simulink model "Delta_Model_Separate"  (R2023a)
settings: Solver=VariableStepAuto  StartTime=0.0  StopTime=10.0  RelTol=1e-3
values from neighbouring files (symbols this model uses):
  coord = [start_coord carry_coord end_coord]    [calculations.m]
  dl = 0.04    [calculations.m]
  l1 = 1    [calculations.m]
  l2 = 3    [calculations.m]
  phi0 = acos((l1+r0-re)/l2)    [calculations.m]
  r0 = 1    [calculations.m]
  re = 0.2    [calculations.m]
  result_t = [start_t carry_t end_t]    [calculations.m]
undefined symbols (not defined in the file or in its folder): B, m1_1, Spline, X, Y, Z
libraries: sm_lib x109, nesl_utility x10, robotcorelib x1
(part 4 of 4)

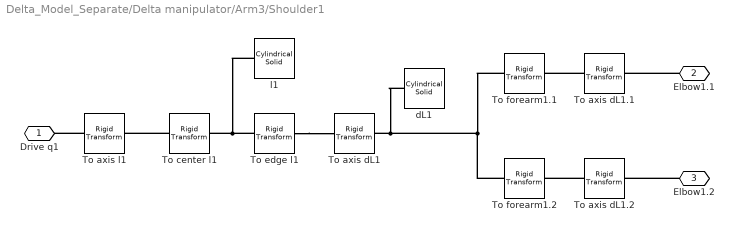
== system Delta_Model_Separate/Delta manipulator/Arm3/Shoulder1 ==
  To axis dL1 : sm_lib/Frames and Transforms/Rigid Transform  TranslationMethod=None  TranslationStandardOffset=0  TranslationStandardOffsetUnits=m  TranslationStandardAxis=+Z  TranslationCartesianOffset=[r0 0 0]  TranslationCartesianOffsetUnits=m  TranslationROffset=0  TranslationROffsetUnits=m  TranslationZOffset=0  TranslationZOffsetUnits=m  TranslationThetaOffset=0  TranslationThetaOffsetUnits=deg  RotationMethod=StandardAxis  RotationAngleUnits=rad  RotationStandardAxis=+Y  RotationAngle=pi/2  RotationArbitraryAxis=[0 0 1]  FollAlignAxisA=+X  BaseAlignAxisA=+Y  FollAlignAxisB=+Y  BaseAlignAxisB=+Z  RotationSequenceAxes=FollowerAxes  RotationSequence=XYX  RotationSequenceAngles=[0 0 0]  RotationSequenceAnglesUnits=deg  RotationMatrix=[1 0 0; 0 1 0; 0 0 1]  Quaternion=[1 0 0 0]
  To axis dL1.1 : sm_lib/Frames and Transforms/Rigid Transform  TranslationMethod=None  TranslationStandardOffset=0  TranslationStandardOffsetUnits=m  TranslationStandardAxis=+Z  TranslationCartesianOffset=[r0 0 0]  TranslationCartesianOffsetUnits=m  TranslationROffset=0  TranslationROffsetUnits=m  TranslationZOffset=0  TranslationZOffsetUnits=m  TranslationThetaOffset=0  TranslationThetaOffsetUnits=deg  RotationMethod=StandardAxis  RotationAngleUnits=rad  RotationStandardAxis=-Y  RotationAngle=pi/2  RotationArbitraryAxis=[0 0 1]  FollAlignAxisA=+X  BaseAlignAxisA=+Y  FollAlignAxisB=+Y  BaseAlignAxisB=+Z  RotationSequenceAxes=FollowerAxes  RotationSequence=XYX  RotationSequenceAngles=[0 0 0]  RotationSequenceAnglesUnits=deg  RotationMatrix=[1 0 0; 0 1 0; 0 0 1]  Quaternion=[1 0 0 0]
  To axis dL1.2 : sm_lib/Frames and Transforms/Rigid Transform  TranslationMethod=None  TranslationStandardOffset=0  TranslationStandardOffsetUnits=m  TranslationStandardAxis=+Z  TranslationCartesianOffset=[r0 0 0]  TranslationCartesianOffsetUnits=m  TranslationROffset=0  TranslationROffsetUnits=m  TranslationZOffset=0  TranslationZOffsetUnits=m  TranslationThetaOffset=0  TranslationThetaOffsetUnits=deg  RotationMethod=StandardAxis  RotationAngleUnits=rad  RotationStandardAxis=-Y  RotationAngle=pi/2  RotationArbitraryAxis=[0 0 1]  FollAlignAxisA=+X  BaseAlignAxisA=+Y  FollAlignAxisB=+Y  BaseAlignAxisB=+Z  RotationSequenceAxes=FollowerAxes  RotationSequence=XYX  RotationSequenceAngles=[0 0 0]  RotationSequenceAnglesUnits=deg  RotationMatrix=[1 0 0; 0 1 0; 0 0 1]  Quaternion=[1 0 0 0]
  To axis l1 : sm_lib/Frames and Transforms/Rigid Transform  TranslationMethod=None  TranslationStandardOffset=0  TranslationStandardOffsetUnits=m  TranslationStandardAxis=+Z  TranslationCartesianOffset=[r0 0 0]  TranslationCartesianOffsetUnits=m  TranslationROffset=0  TranslationROffsetUnits=m  TranslationZOffset=0  TranslationZOffsetUnits=m  TranslationThetaOffset=0  TranslationThetaOffsetUnits=deg  RotationMethod=StandardAxis  RotationAngleUnits=deg  RotationStandardAxis=+Y  RotationAngle=90  RotationArbitraryAxis=[0 0 1]  FollAlignAxisA=+X  BaseAlignAxisA=+Y  FollAlignAxisB=+Y  BaseAlignAxisB=+Z  RotationSequenceAxes=FollowerAxes  RotationSequence=XYX  RotationSequenceAngles=[0 0 0]  RotationSequenceAnglesUnits=deg  RotationMatrix=[1 0 0; 0 1 0; 0 0 1]  Quaternion=[1 0 0 0]
  To center l1 : sm_lib/Frames and Transforms/Rigid Transform  TranslationMethod=Cartesian  TranslationStandardOffset=0  TranslationStandardOffsetUnits=m  TranslationStandardAxis=+Z  TranslationCartesianOffset=[0 0 l1/2]  TranslationCartesianOffsetUnits=m  TranslationROffset=0  TranslationROffsetUnits=m  TranslationZOffset=0  TranslationZOffsetUnits=m  TranslationThetaOffset=0  TranslationThetaOffsetUnits=deg  RotationMethod=None  RotationAngleUnits=deg  RotationStandardAxis=+Y  RotationAngle=90  RotationArbitraryAxis=[0 0 1]  FollAlignAxisA=+X  BaseAlignAxisA=+Y  FollAlignAxisB=+Y  BaseAlignAxisB=+Z  RotationSequenceAxes=FollowerAxes  RotationSequence=XYX  RotationSequenceAngles=[0 0 0]  RotationSequenceAnglesUnits=deg  RotationMatrix=[1 0 0; 0 1 0; 0 0 1]  Quaternion=[1 0 0 0]
  To edge l1 : sm_lib/Frames and Transforms/Rigid Transform  TranslationMethod=Cartesian  TranslationStandardOffset=0  TranslationStandardOffsetUnits=m  TranslationStandardAxis=+Z  TranslationCartesianOffset=[0 0 l1/2]  TranslationCartesianOffsetUnits=m  TranslationROffset=0  TranslationROffsetUnits=m  TranslationZOffset=0  TranslationZOffsetUnits=m  TranslationThetaOffset=0  TranslationThetaOffsetUnits=deg  RotationMethod=None  RotationAngleUnits=deg  RotationStandardAxis=+Y  RotationAngle=90  RotationArbitraryAxis=[0 0 1]  FollAlignAxisA=+X  BaseAlignAxisA=+Y  FollAlignAxisB=+Y  BaseAlignAxisB=+Z  RotationSequenceAxes=FollowerAxes  RotationSequence=XYX  RotationSequenceAngles=[0 0 0]  RotationSequenceAnglesUnits=deg  RotationMatrix=[1 0 0; 0 1 0; 0 0 1]  Quaternion=[1 0 0 0]
  "To forearm1.1 " : sm_lib/Frames and Transforms/Rigid Transform  TranslationMethod=Cartesian  TranslationStandardOffset=0  TranslationStandardOffsetUnits=m  TranslationStandardAxis=+Z  TranslationCartesianOffset=[0 0 dl/2]  TranslationCartesianOffsetUnits=m  TranslationROffset=0  TranslationROffsetUnits=m  TranslationZOffset=0  TranslationZOffsetUnits=m  TranslationThetaOffset=0  TranslationThetaOffsetUnits=deg  RotationMethod=None  RotationAngleUnits=deg  RotationStandardAxis=+Y  RotationAngle=90  RotationArbitraryAxis=[0 0 1]  FollAlignAxisA=+X  BaseAlignAxisA=+Y  FollAlignAxisB=+Y  BaseAlignAxisB=+Z  RotationSequenceAxes=FollowerAxes  RotationSequence=XYX  RotationSequenceAngles=[0 0 0]  RotationSequenceAnglesUnits=deg  RotationMatrix=[1 0 0; 0 1 0; 0 0 1]  Quaternion=[1 0 0 0]
  To forearm1.2 : sm_lib/Frames and Transforms/Rigid Transform  TranslationMethod=Cartesian  TranslationStandardOffset=0  TranslationStandardOffsetUnits=m  TranslationStandardAxis=+Z  TranslationCartesianOffset=[0 0 -dl/2]  TranslationCartesianOffsetUnits=m  TranslationROffset=0  TranslationROffsetUnits=m  TranslationZOffset=0  TranslationZOffsetUnits=m  TranslationThetaOffset=0  TranslationThetaOffsetUnits=deg  RotationMethod=None  RotationAngleUnits=deg  RotationStandardAxis=+Y  RotationAngle=90  RotationArbitraryAxis=[0 0 1]  FollAlignAxisA=+X  BaseAlignAxisA=+Y  FollAlignAxisB=+Y  BaseAlignAxisB=+Z  RotationSequenceAxes=FollowerAxes  RotationSequence=XYX  RotationSequenceAngles=[0 0 0]  RotationSequenceAnglesUnits=deg  RotationMatrix=[1 0 0; 0 1 0; 0 0 1]  Quaternion=[1 0 0 0]
  dL1 : sm_lib/Body Elements/Cylindrical Solid  GraphicAmbientColor=[0.15 0.15 0.15 1.0]  BasedOnType=Density  CenterOfMass=[0 0 0]  CenterOfMassUnits=m  GraphicDiffuseColor=[0.2 0.6 1.0]  CylinderLength=dl  CylinderLengthUnits=m  CylinderRadius=rdl  CylinderRadiusUnits=m  Density=1000  DensityUnits=kg/m^3  DoExposeReferenceFrame=on  GraphicEmissiveColor=[0.0 0.0 0.0 1.0]  ExportEntireGeometry=off  SerializedFrames=<Frames/>  MarkerShape=Sphere  MarkerSize=10  GraphicType=FromGeometry  InertiaType=CalculateFromGeometry  Mass=m1_1  MassUnits=kg  MomentsOfInertia=[1 1 1]  MomentsOfInertiaUnits=kg*m^2  GraphicOpacity=1.0  ProductsOfInertia=[0 0 0]  ProductsOfInertiaUnits=kg*m^2  GraphicShininess=75  GraphicSpecularColor=[0.5 0.5 0.5 1.0]  GraphicVisPropType=SimpleVisualProperties
  l1 : sm_lib/Body Elements/Cylindrical Solid  GraphicAmbientColor=[0.15 0.15 0.15 1.0]  BasedOnType=Density  CenterOfMass=[0 0 0]  CenterOfMassUnits=m  GraphicDiffuseColor=[0.2 0.6 1.0]  CylinderLength=l1  CylinderLengthUnits=m  CylinderRadius=rl1  CylinderRadiusUnits=m  Density=1000  DensityUnits=kg/m^3  DoExposeReferenceFrame=on  GraphicEmissiveColor=[0.0 0.0 0.0 1.0]  ExportEntireGeometry=off  SerializedFrames=<Frames/>  MarkerShape=Sphere  MarkerSize=10  GraphicType=FromGeometry  InertiaType=CalculateFromGeometry  Mass=m1_1  MassUnits=kg  MomentsOfInertia=[1 1 1]  MomentsOfInertiaUnits=kg*m^2  GraphicOpacity=1.0  ProductsOfInertia=[0 0 0]  ProductsOfInertiaUnits=kg*m^2  GraphicShininess=75  GraphicSpecularColor=[0.5 0.5 0.5 1.0]  GraphicVisPropType=SimpleVisualProperties
  Drive q1 : PMIOPort  Side=Left
  Elbow1.1 : PMIOPort  Port=2  Side=Right
  Elbow1.2 : PMIOPort  Port=3  Side=Right
  connections:
  l1/RConn1 -- To edge l1/LConn1 -- To center l1/RConn1
  To center l1/LConn1 -- To axis l1/RConn1
  To axis l1/LConn1 -- Drive q1/RConn1
  "To forearm1.1 "/LConn1 -- dL1/RConn1 -- To axis dL1/RConn1 -- To forearm1.2/LConn1
  To edge l1/RConn1 -- To axis dL1/LConn1
  To axis dL1.1/LConn1 -- "To forearm1.1 "/RConn1
  To axis dL1.2/LConn1 -- To forearm1.2/RConn1
  Elbow1.1/RConn1 -- To axis dL1.1/RConn1
  Elbow1.2/RConn1 -- To axis dL1.2/RConn1

== matlab function Delta_Model_Separate/IKINE/MATLAB Function5 ==
  data: l1 input; condition output; l1 output; l2 output; xei output; yei output; zei output; xp output; yp output; zp output; al output; l2 input; xei input; yei input; zei input; xp input; yp input; zp input; a output; b output; c output; al input
function [condition, l1, l2, xei, yei, zei, xp, yp, zp, al, a, b, c] = condition(l1, l2, xei, yei, zei, xp, yp, zp, al)
a = 2*l2^2*xei^2 + 2*l2^2*xp^2 + 2*l2^2*yei^2 + 2*l2^2*yp^2 + 2*l1^2*zei^2 + 2*l2^2*zei^2 + 2*l1^2*zp^2 + 2*l2^2*zp^2 - 6*xei^2*xp^2 - 2*xei^2*yei^2 - 2*xei^2*yp^2 - 2*xp^2*yei^2 - 2*xp^2*yp^2 - 2*xei^2*zei^2 - 2*xei^2*zp^2 - 2*xp^2*zei^2 - 6*yei^2*yp^2 - 2*xp^2*zp^2 - 2*yei^2*zei^2 - 2*yei^2*zp^2 - 2*yp^2*zei^2 - 2*yp^2*zp^2 - 6*zei^2*zp^2 + 4*xei*xp^3 + 4*xei^3*xp + 4*yei*yp^3 + 4*yei^3*yp + 4*zei*zp^3 + 4*zei^3*zp - l1^4 - l2^4 - xei^4 - xp^4 - yei^4 - yp^4 - zei^4 - zp^4 + 2*l1^2*l2^2 - 4*l2^2*xei*xp - 4*l2^2*yei*yp - 4*l1^2*zei*zp - 4*l2^2*zei*zp + 2*l1^2*xei^2*cos(2*al) + 2*l1^2*xp^2*cos(2*al) - 2*l1^2*yei^2*cos(2*al) - 2*l1^2*yp^2*cos(2*al) + 4*xei*xp*yei^2 + 4*xei*xp*yp^2 + 4*xei*xp*zei^2 + 4*xei^2*yei*yp + 4*xei*xp*zp^2 + 4*xp^2*yei*yp + 4*yei*yp*zei^2 + 4*xei^2*zei*zp + 4*yei*yp*zp^2 + 4*xp^2*zei*zp + 4*yei^2*zei*zp + 4*yp^2*zei*zp - 4*l1^2*xei*xp*cos(2*al) + 4*l1^2*yei*yp*cos(2*al) - 8*xei*xp*yei*yp - 8*xei*xp*zei*zp - 8*yei*yp*zei*zp + 4*l1^2*xei*yei*sin(2*al) - 4*l1^2*xei*yp*sin(2*al) - 4*l1^2*xp*yei*sin(2*al) + 4*l1^2*xp*yp*sin(2*al);
b = xei^2*cos(al)^2 - 2*zei*zp + xp^2*cos(al)^2 + yei^2*sin(al)^2 + yp^2*sin(al)^2 + zei^2 + zp^2 - 2*xei*xp*cos(al)^2 + xei*yei*sin(2*al) - xei*yp*sin(2*al) - xp*yei*sin(2*al) + xp*yp*sin(2*al) - 2*yei*yp*sin(al)^2;
c = xei*cos(al) - xp*cos(al) + yei*sin(al) - yp*sin(al);
condition = a >= 0 & b ~= 0 & c ~= 0;
end

== matlab function Delta_Model_Separate/IKINE/MATLAB Function6 ==
  data: q output; l1 input; l2 input; xei input; yei input; zei input; xp input; yp input; zp input; al input; a input; b input; c input
function q = q(l1, l2, xei, yei, zei, xp, yp, zp, al, a, b, c)
k = 0;
q = zeros(1,4);
q(1) = asin((zp^3*abs(c)*abs(l1) - zei^3*abs(c)*abs(l1) - l1^2*zei*abs(c)*abs(l1) + l2^2*zei*abs(c)*abs(l1) + l1^2*zp*abs(c)*abs(l1) - l2^2*zp*abs(c)*abs(l1) - xei^2*zei*abs(c)*abs(l1) + xei^2*zp*abs(c)*abs(l1) - xp^2*zei*abs(c)*abs(l1) + xp^2*zp*abs(c)*abs(l1) - yei^2*zei*abs(c)*abs(l1) + yei^2*zp*abs(c)*abs(l1) - yp^2*zei*abs(c)*abs(l1) + yp^2*zp*abs(c)*abs(l1) - 3*zei*zp^2*abs(c)*abs(l1) + 3*zei^2*zp*abs(c)*abs(l1) + a^(1/2)*l1*xei^2*cos(al)^2 + a^(1/2)*l1*xp^2*cos(al)^2 + a^(1/2)*l1*yei^2*sin(al)^2 + a^(1/2)*l1*yp^2*sin(al)^2 + 2*xei*xp*zei*abs(c)*abs(l1) - 2*xei*xp*zp*abs(c)*abs(l1) + 2*yei*yp*zei*abs(c)*abs(l1) - 2*yei*yp*zp*abs(c)*abs(l1) - 2*a^(1/2)*l1*xei*xp*cos(al)^2 + a^(1/2)*l1*xei*yei*sin(2*al) - a^(1/2)*l1*xei*yp*sin(2*al) - a^(1/2)*l1*xp*yei*sin(2*al) + a^(1/2)*l1*xp*yp*sin(2*al) - 2*a^(1/2)*l1*yei*yp*sin(al)^2)/(2*b*l1*abs(c)*abs(l1))) + 2*k*pi;
q(2) = 2*k*pi - asin((zei^3*abs(c)*abs(l1) - zp^3*abs(c)*abs(l1) + l1^2*zei*abs(c)*abs(l1) - l2^2*zei*abs(c)*abs(l1) - l1^2*zp*abs(c)*abs(l1) + l2^2*zp*abs(c)*abs(l1) + xei^2*zei*abs(c)*abs(l1) - xei^2*zp*abs(c)*abs(l1) + xp^2*zei*abs(c)*abs(l1) - xp^2*zp*abs(c)*abs(l1) + yei^2*zei*abs(c)*abs(l1) - yei^2*zp*abs(c)*abs(l1) + yp^2*zei*abs(c)*abs(l1) - yp^2*zp*abs(c)*abs(l1) + 3*zei*zp^2*abs(c)*abs(l1) - 3*zei^2*zp*abs(c)*abs(l1) + a^(1/2)*l1*xei^2*cos(al)^2 + a^(1/2)*l1*xp^2*cos(al)^2 + a^(1/2)*l1*yei^2*sin(al)^2 + a^(1/2)*l1*yp^2*sin(al)^2 - 2*xei*xp*zei*abs(c)*abs(l1) + 2*xei*xp*zp*abs(c)*abs(l1) - 2*yei*yp*zei*abs(c)*abs(l1) + 2*yei*yp*zp*abs(c)*abs(l1) - 2*a^(1/2)*l1*xei*xp*cos(al)^2 + a^(1/2)*l1*xei*yei*sin(2*al) - a^(1/2)*l1*xei*yp*sin(2*al) - a^(1/2)*l1*xp*yei*sin(2*al) + a^(1/2)*l1*xp*yp*sin(2*al) - 2*a^(1/2)*l1*yei*yp*sin(al)^2)/(2*b*l1*abs(c)*abs(l1)));
q(3) = pi + asin((zei^3*abs(c)*abs(l1) - zp^3*abs(c)*abs(l1) + l1^2*zei*abs(c)*abs(l1) - l2^2*zei*abs(c)*abs(l1) - l1^2*zp*abs(c)*abs(l1) + l2^2*zp*abs(c)*abs(l1) + xei^2*zei*abs(c)*abs(l1) - xei^2*zp*abs(c)*abs(l1) + xp^2*zei*abs(c)*abs(l1) - xp^2*zp*abs(c)*abs(l1) + yei^2*zei*abs(c)*abs(l1) - yei^2*zp*abs(c)*abs(l1) + yp^2*zei*abs(c)*abs(l1) - yp^2*zp*abs(c)*abs(l1) + 3*zei*zp^2*abs(c)*abs(l1) - 3*zei^2*zp*abs(c)*abs(l1) + a^(1/2)*l1*xei^2*cos(al)^2 + a^(1/2)*l1*xp^2*cos(al)^2 + a^(1/2)*l1*yei^2*sin(al)^2 + a^(1/2)*l1*yp^2*sin(al)^2 - 2*xei*xp*zei*abs(c)*abs(l1) + 2*xei*xp*zp*abs(c)*abs(l1) - 2*yei*yp*zei*abs(c)*abs(l1) + 2*yei*yp*zp*abs(c)*abs(l1) - 2*a^(1/2)*l1*xei*xp*cos(al)^2 + a^(1/2)*l1*xei*yei*sin(2*al) - a^(1/2)*l1*xei*yp*sin(2*al) - a^(1/2)*l1*xp*yei*sin(2*al) + a^(1/2)*l1*xp*yp*sin(2*al) - 2*a^(1/2)*l1*yei*yp*sin(al)^2)/(2*b*l1*abs(c)*abs(l1))) + 2*k*pi;
q(4) = pi - asin((zp^3*abs(c)*abs(l1) - zei^3*abs(c)*abs(l1) - l1^2*zei*abs(c)*abs(l1) + l2^2*zei*abs(c)*abs(l1) + l1^2*zp*abs(c)*abs(l1) - l2^2*zp*abs(c)*abs(l1) - xei^2*zei*abs(c)*abs(l1) + xei^2*zp*abs(c)*abs(l1) - xp^2*zei*abs(c)*abs(l1) + xp^2*zp*abs(c)*abs(l1) - yei^2*zei*abs(c)*abs(l1) + yei^2*zp*abs(c)*abs(l1) - yp^2*zei*abs(c)*abs(l1) + yp^2*zp*abs(c)*abs(l1) - 3*zei*zp^2*abs(c)*abs(l1) + 3*zei^2*zp*abs(c)*abs(l1) + a^(1/2)*l1*xei^2*cos(al)^2 + a^(1/2)*l1*xp^2*cos(al)^2 + a^(1/2)*l1*yei^2*sin(al)^2 + a^(1/2)*l1*yp^2*sin(al)^2 + 2*xei*xp*zei*abs(c)*abs(l1) - 2*xei*xp*zp*abs(c)*abs(l1) + 2*yei*yp*zei*abs(c)*abs(l1) - 2*yei*yp*zp*abs(c)*abs(l1) - 2*a^(1/2)*l1*xei*xp*cos(al)^2 + a^(1/2)*l1*xei*yei*sin(2*al) - a^(1/2)*l1*xei*yp*sin(2*al) - a^(1/2)*l1*xp*yei*sin(2*al) + a^(1/2)*l1*xp*yp*sin(2*al) - 2*a^(1/2)*l1*yei*yp*sin(al)^2)/(2*b*l1*abs(c)*abs(l1))) + 2*k*pi;
end

== matlab function Delta_Model_Separate/IKINE/MATLAB Function7 ==
  data: l1 input; l2 input; q output; xei input; yei input; zei input; xp input; yp input; zp input; al input; a input; b input; c input
function q = q(l1, l2, xei, yei, zei, xp, yp, zp, al, a, b, c)
k = 0;
q = zeros(1,4);
q(1) = asin((zp^3*abs(c)*abs(l1) - zei^3*abs(c)*abs(l1) - l1^2*zei*abs(c)*abs(l1) + l2^2*zei*abs(c)*abs(l1) + l1^2*zp*abs(c)*abs(l1) - l2^2*zp*abs(c)*abs(l1) - xei^2*zei*abs(c)*abs(l1) + xei^2*zp*abs(c)*abs(l1) - xp^2*zei*abs(c)*abs(l1) + xp^2*zp*abs(c)*abs(l1) - yei^2*zei*abs(c)*abs(l1) + yei^2*zp*abs(c)*abs(l1) - yp^2*zei*abs(c)*abs(l1) + yp^2*zp*abs(c)*abs(l1) - 3*zei*zp^2*abs(c)*abs(l1) + 3*zei^2*zp*abs(c)*abs(l1) + a^(1/2)*l1*xei^2*cos(al)^2 + a^(1/2)*l1*xp^2*cos(al)^2 + a^(1/2)*l1*yei^2*sin(al)^2 + a^(1/2)*l1*yp^2*sin(al)^2 + 2*xei*xp*zei*abs(c)*abs(l1) - 2*xei*xp*zp*abs(c)*abs(l1) + 2*yei*yp*zei*abs(c)*abs(l1) - 2*yei*yp*zp*abs(c)*abs(l1) - 2*a^(1/2)*l1*xei*xp*cos(al)^2 + a^(1/2)*l1*xei*yei*sin(2*al) - a^(1/2)*l1*xei*yp*sin(2*al) - a^(1/2)*l1*xp*yei*sin(2*al) + a^(1/2)*l1*xp*yp*sin(2*al) - 2*a^(1/2)*l1*yei*yp*sin(al)^2)/(2*b*l1*abs(c)*abs(l1))) + 2*k*pi;
q(2) = 2*k*pi - asin((zei^3*abs(c)*abs(l1) - zp^3*abs(c)*abs(l1) + l1^2*zei*abs(c)*abs(l1) - l2^2*zei*abs(c)*abs(l1) - l1^2*zp*abs(c)*abs(l1) + l2^2*zp*abs(c)*abs(l1) + xei^2*zei*abs(c)*abs(l1) - xei^2*zp*abs(c)*abs(l1) + xp^2*zei*abs(c)*abs(l1) - xp^2*zp*abs(c)*abs(l1) + yei^2*zei*abs(c)*abs(l1) - yei^2*zp*abs(c)*abs(l1) + yp^2*zei*abs(c)*abs(l1) - yp^2*zp*abs(c)*abs(l1) + 3*zei*zp^2*abs(c)*abs(l1) - 3*zei^2*zp*abs(c)*abs(l1) + a^(1/2)*l1*xei^2*cos(al)^2 + a^(1/2)*l1*xp^2*cos(al)^2 + a^(1/2)*l1*yei^2*sin(al)^2 + a^(1/2)*l1*yp^2*sin(al)^2 - 2*xei*xp*zei*abs(c)*abs(l1) + 2*xei*xp*zp*abs(c)*abs(l1) - 2*yei*yp*zei*abs(c)*abs(l1) + 2*yei*yp*zp*abs(c)*abs(l1) - 2*a^(1/2)*l1*xei*xp*cos(al)^2 + a^(1/2)*l1*xei*yei*sin(2*al) - a^(1/2)*l1*xei*yp*sin(2*al) - a^(1/2)*l1*xp*yei*sin(2*al) + a^(1/2)*l1*xp*yp*sin(2*al) - 2*a^(1/2)*l1*yei*yp*sin(al)^2)/(2*b*l1*abs(c)*abs(l1)));
q(3) = pi + asin((zei^3*abs(c)*abs(l1) - zp^3*abs(c)*abs(l1) + l1^2*zei*abs(c)*abs(l1) - l2^2*zei*abs(c)*abs(l1) - l1^2*zp*abs(c)*abs(l1) + l2^2*zp*abs(c)*abs(l1) + xei^2*zei*abs(c)*abs(l1) - xei^2*zp*abs(c)*abs(l1) + xp^2*zei*abs(c)*abs(l1) - xp^2*zp*abs(c)*abs(l1) + yei^2*zei*abs(c)*abs(l1) - yei^2*zp*abs(c)*abs(l1) + yp^2*zei*abs(c)*abs(l1) - yp^2*zp*abs(c)*abs(l1) + 3*zei*zp^2*abs(c)*abs(l1) - 3*zei^2*zp*abs(c)*abs(l1) + a^(1/2)*l1*xei^2*cos(al)^2 + a^(1/2)*l1*xp^2*cos(al)^2 + a^(1/2)*l1*yei^2*sin(al)^2 + a^(1/2)*l1*yp^2*sin(al)^2 - 2*xei*xp*zei*abs(c)*abs(l1) + 2*xei*xp*zp*abs(c)*abs(l1) - 2*yei*yp*zei*abs(c)*abs(l1) + 2*yei*yp*zp*abs(c)*abs(l1) - 2*a^(1/2)*l1*xei*xp*cos(al)^2 + a^(1/2)*l1*xei*yei*sin(2*al) - a^(1/2)*l1*xei*yp*sin(2*al) - a^(1/2)*l1*xp*yei*sin(2*al) + a^(1/2)*l1*xp*yp*sin(2*al) - 2*a^(1/2)*l1*yei*yp*sin(al)^2)/(2*b*l1*abs(c)*abs(l1))) + 2*k*pi;
q(4) = pi - asin((zp^3*abs(c)*abs(l1) - zei^3*abs(c)*abs(l1) - l1^2*zei*abs(c)*abs(l1) + l2^2*zei*abs(c)*abs(l1) + l1^2*zp*abs(c)*abs(l1) - l2^2*zp*abs(c)*abs(l1) - xei^2*zei*abs(c)*abs(l1) + xei^2*zp*abs(c)*abs(l1) - xp^2*zei*abs(c)*abs(l1) + xp^2*zp*abs(c)*abs(l1) - yei^2*zei*abs(c)*abs(l1) + yei^2*zp*abs(c)*abs(l1) - yp^2*zei*abs(c)*abs(l1) + yp^2*zp*abs(c)*abs(l1) - 3*zei*zp^2*abs(c)*abs(l1) + 3*zei^2*zp*abs(c)*abs(l1) + a^(1/2)*l1*xei^2*cos(al)^2 + a^(1/2)*l1*xp^2*cos(al)^2 + a^(1/2)*l1*yei^2*sin(al)^2 + a^(1/2)*l1*yp^2*sin(al)^2 + 2*xei*xp*zei*abs(c)*abs(l1) - 2*xei*xp*zp*abs(c)*abs(l1) + 2*yei*yp*zei*abs(c)*abs(l1) - 2*yei*yp*zp*abs(c)*abs(l1) - 2*a^(1/2)*l1*xei*xp*cos(al)^2 + a^(1/2)*l1*xei*yei*sin(2*al) - a^(1/2)*l1*xei*yp*sin(2*al) - a^(1/2)*l1*xp*yei*sin(2*al) + a^(1/2)*l1*xp*yp*sin(2*al) - 2*a^(1/2)*l1*yei*yp*sin(al)^2)/(2*b*l1*abs(c)*abs(l1))) + 2*k*pi;
end

== matlab function Delta_Model_Separate/IKINE/MATLAB Function8 ==
  data: l1 input; l2 input; q output; xei input; yei input; zei input; xp input; yp input; zp input; al input; a input; b input; c input
function q = q(l1, l2, xei, yei, zei, xp, yp, zp, al, a, b, c)
k = 0;
q = zeros(1,4);
q(1) = asin((zp^3*abs(c)*abs(l1) - zei^3*abs(c)*abs(l1) - l1^2*zei*abs(c)*abs(l1) + l2^2*zei*abs(c)*abs(l1) + l1^2*zp*abs(c)*abs(l1) - l2^2*zp*abs(c)*abs(l1) - xei^2*zei*abs(c)*abs(l1) + xei^2*zp*abs(c)*abs(l1) - xp^2*zei*abs(c)*abs(l1) + xp^2*zp*abs(c)*abs(l1) - yei^2*zei*abs(c)*abs(l1) + yei^2*zp*abs(c)*abs(l1) - yp^2*zei*abs(c)*abs(l1) + yp^2*zp*abs(c)*abs(l1) - 3*zei*zp^2*abs(c)*abs(l1) + 3*zei^2*zp*abs(c)*abs(l1) + a^(1/2)*l1*xei^2*cos(al)^2 + a^(1/2)*l1*xp^2*cos(al)^2 + a^(1/2)*l1*yei^2*sin(al)^2 + a^(1/2)*l1*yp^2*sin(al)^2 + 2*xei*xp*zei*abs(c)*abs(l1) - 2*xei*xp*zp*abs(c)*abs(l1) + 2*yei*yp*zei*abs(c)*abs(l1) - 2*yei*yp*zp*abs(c)*abs(l1) - 2*a^(1/2)*l1*xei*xp*cos(al)^2 + a^(1/2)*l1*xei*yei*sin(2*al) - a^(1/2)*l1*xei*yp*sin(2*al) - a^(1/2)*l1*xp*yei*sin(2*al) + a^(1/2)*l1*xp*yp*sin(2*al) - 2*a^(1/2)*l1*yei*yp*sin(al)^2)/(2*b*l1*abs(c)*abs(l1))) + 2*k*pi;
q(2) = 2*k*pi - asin((zei^3*abs(c)*abs(l1) - zp^3*abs(c)*abs(l1) + l1^2*zei*abs(c)*abs(l1) - l2^2*zei*abs(c)*abs(l1) - l1^2*zp*abs(c)*abs(l1) + l2^2*zp*abs(c)*abs(l1) + xei^2*zei*abs(c)*abs(l1) - xei^2*zp*abs(c)*abs(l1) + xp^2*zei*abs(c)*abs(l1) - xp^2*zp*abs(c)*abs(l1) + yei^2*zei*abs(c)*abs(l1) - yei^2*zp*abs(c)*abs(l1) + yp^2*zei*abs(c)*abs(l1) - yp^2*zp*abs(c)*abs(l1) + 3*zei*zp^2*abs(c)*abs(l1) - 3*zei^2*zp*abs(c)*abs(l1) + a^(1/2)*l1*xei^2*cos(al)^2 + a^(1/2)*l1*xp^2*cos(al)^2 + a^(1/2)*l1*yei^2*sin(al)^2 + a^(1/2)*l1*yp^2*sin(al)^2 - 2*xei*xp*zei*abs(c)*abs(l1) + 2*xei*xp*zp*abs(c)*abs(l1) - 2*yei*yp*zei*abs(c)*abs(l1) + 2*yei*yp*zp*abs(c)*abs(l1) - 2*a^(1/2)*l1*xei*xp*cos(al)^2 + a^(1/2)*l1*xei*yei*sin(2*al) - a^(1/2)*l1*xei*yp*sin(2*al) - a^(1/2)*l1*xp*yei*sin(2*al) + a^(1/2)*l1*xp*yp*sin(2*al) - 2*a^(1/2)*l1*yei*yp*sin(al)^2)/(2*b*l1*abs(c)*abs(l1)));
q(3) = pi + asin((zei^3*abs(c)*abs(l1) - zp^3*abs(c)*abs(l1) + l1^2*zei*abs(c)*abs(l1) - l2^2*zei*abs(c)*abs(l1) - l1^2*zp*abs(c)*abs(l1) + l2^2*zp*abs(c)*abs(l1) + xei^2*zei*abs(c)*abs(l1) - xei^2*zp*abs(c)*abs(l1) + xp^2*zei*abs(c)*abs(l1) - xp^2*zp*abs(c)*abs(l1) + yei^2*zei*abs(c)*abs(l1) - yei^2*zp*abs(c)*abs(l1) + yp^2*zei*abs(c)*abs(l1) - yp^2*zp*abs(c)*abs(l1) + 3*zei*zp^2*abs(c)*abs(l1) - 3*zei^2*zp*abs(c)*abs(l1) + a^(1/2)*l1*xei^2*cos(al)^2 + a^(1/2)*l1*xp^2*cos(al)^2 + a^(1/2)*l1*yei^2*sin(al)^2 + a^(1/2)*l1*yp^2*sin(al)^2 - 2*xei*xp*zei*abs(c)*abs(l1) + 2*xei*xp*zp*abs(c)*abs(l1) - 2*yei*yp*zei*abs(c)*abs(l1) + 2*yei*yp*zp*abs(c)*abs(l1) - 2*a^(1/2)*l1*xei*xp*cos(al)^2 + a^(1/2)*l1*xei*yei*sin(2*al) - a^(1/2)*l1*xei*yp*sin(2*al) - a^(1/2)*l1*xp*yei*sin(2*al) + a^(1/2)*l1*xp*yp*sin(2*al) - 2*a^(1/2)*l1*yei*yp*sin(al)^2)/(2*b*l1*abs(c)*abs(l1))) + 2*k*pi;
q(4) = pi - asin((zp^3*abs(c)*abs(l1) - zei^3*abs(c)*abs(l1) - l1^2*zei*abs(c)*abs(l1) + l2^2*zei*abs(c)*abs(l1) + l1^2*zp*abs(c)*abs(l1) - l2^2*zp*abs(c)*abs(l1) - xei^2*zei*abs(c)*abs(l1) + xei^2*zp*abs(c)*abs(l1) - xp^2*zei*abs(c)*abs(l1) + xp^2*zp*abs(c)*abs(l1) - yei^2*zei*abs(c)*abs(l1) + yei^2*zp*abs(c)*abs(l1) - yp^2*zei*abs(c)*abs(l1) + yp^2*zp*abs(c)*abs(l1) - 3*zei*zp^2*abs(c)*abs(l1) + 3*zei^2*zp*abs(c)*abs(l1) + a^(1/2)*l1*xei^2*cos(al)^2 + a^(1/2)*l1*xp^2*cos(al)^2 + a^(1/2)*l1*yei^2*sin(al)^2 + a^(1/2)*l1*yp^2*sin(al)^2 + 2*xei*xp*zei*abs(c)*abs(l1) - 2*xei*xp*zp*abs(c)*abs(l1) + 2*yei*yp*zei*abs(c)*abs(l1) - 2*yei*yp*zp*abs(c)*abs(l1) - 2*a^(1/2)*l1*xei*xp*cos(al)^2 + a^(1/2)*l1*xei*yei*sin(2*al) - a^(1/2)*l1*xei*yp*sin(2*al) - a^(1/2)*l1*xp*yei*sin(2*al) + a^(1/2)*l1*xp*yp*sin(2*al) - 2*a^(1/2)*l1*yei*yp*sin(al)^2)/(2*b*l1*abs(c)*abs(l1))) + 2*k*pi;
end

== matlab function Delta_Model_Separate/IKINE/MATLAB Function2 ==
  data: r0 input; xe1 output; re input; xe input; ye input; ze input; ye1 output; ze1 output; xp1 output; yp1 output; zp1 output; al1 output; xe2 output; ye2 output; ze2 output; xp2 output; yp2 output; zp2 output; al2 output; xe3 output; ye3 output; ze3 output; xp3 output; yp3 output; zp3 output; al1 input; al2 input; al3 input; al3 output
function [xe1, ye1, ze1, xp1, yp1, zp1, al1, xe2, ye2, ze2, xp2, yp2, zp2, al2, xe3, ye3, ze3, xp3, yp3, zp3, al3] = joint_coordinates(r0, re, xe, ye, ze, al1, al2, al3)
xe1 = xe + re*cos(al1);
ye1 = ye + re*sin(al1);
ze1 = ze;
xp1 = r0*cos(al1);
yp1 = r0*sin(al1);
zp1 = 0;
xe2 = xe + re*cos(al2);
ye2 = ye + re*sin(al2);
ze2 = ze;
xp2 = r0*cos(al2);
yp2 = r0*sin(al2);
zp2 = 0;
xe3 = xe + re*cos(al3);
ye3 = ye + re*sin(al3);
ze3 = ze;
xp3 = r0*cos(al3);
yp3 = r0*sin(al3);
zp3 = 0;
end

== matlab function Delta_Model_Separate/IKINE/MATLAB Function3 ==
  data: l1 input; condition output; l1 output; l2 output; xei output; yei output; zei output; xp output; yp output; zp output; al output; l2 input; xei input; yei input; zei input; xp input; yp input; zp input; a output; b output; c output; al input
function [condition, l1, l2, xei, yei, zei, xp, yp, zp, al, a, b, c] = condition(l1, l2, xei, yei, zei, xp, yp, zp, al)
a = 2*l2^2*xei^2 + 2*l2^2*xp^2 + 2*l2^2*yei^2 + 2*l2^2*yp^2 + 2*l1^2*zei^2 + 2*l2^2*zei^2 + 2*l1^2*zp^2 + 2*l2^2*zp^2 - 6*xei^2*xp^2 - 2*xei^2*yei^2 - 2*xei^2*yp^2 - 2*xp^2*yei^2 - 2*xp^2*yp^2 - 2*xei^2*zei^2 - 2*xei^2*zp^2 - 2*xp^2*zei^2 - 6*yei^2*yp^2 - 2*xp^2*zp^2 - 2*yei^2*zei^2 - 2*yei^2*zp^2 - 2*yp^2*zei^2 - 2*yp^2*zp^2 - 6*zei^2*zp^2 + 4*xei*xp^3 + 4*xei^3*xp + 4*yei*yp^3 + 4*yei^3*yp + 4*zei*zp^3 + 4*zei^3*zp - l1^4 - l2^4 - xei^4 - xp^4 - yei^4 - yp^4 - zei^4 - zp^4 + 2*l1^2*l2^2 - 4*l2^2*xei*xp - 4*l2^2*yei*yp - 4*l1^2*zei*zp - 4*l2^2*zei*zp + 2*l1^2*xei^2*cos(2*al) + 2*l1^2*xp^2*cos(2*al) - 2*l1^2*yei^2*cos(2*al) - 2*l1^2*yp^2*cos(2*al) + 4*xei*xp*yei^2 + 4*xei*xp*yp^2 + 4*xei*xp*zei^2 + 4*xei^2*yei*yp + 4*xei*xp*zp^2 + 4*xp^2*yei*yp + 4*yei*yp*zei^2 + 4*xei^2*zei*zp + 4*yei*yp*zp^2 + 4*xp^2*zei*zp + 4*yei^2*zei*zp + 4*yp^2*zei*zp - 4*l1^2*xei*xp*cos(2*al) + 4*l1^2*yei*yp*cos(2*al) - 8*xei*xp*yei*yp - 8*xei*xp*zei*zp - 8*yei*yp*zei*zp + 4*l1^2*xei*yei*sin(2*al) - 4*l1^2*xei*yp*sin(2*al) - 4*l1^2*xp*yei*sin(2*al) + 4*l1^2*xp*yp*sin(2*al);
b = xei^2*cos(al)^2 - 2*zei*zp + xp^2*cos(al)^2 + yei^2*sin(al)^2 + yp^2*sin(al)^2 + zei^2 + zp^2 - 2*xei*xp*cos(al)^2 + xei*yei*sin(2*al) - xei*yp*sin(2*al) - xp*yei*sin(2*al) + xp*yp*sin(2*al) - 2*yei*yp*sin(al)^2;
c = xei*cos(al) - xp*cos(al) + yei*sin(al) - yp*sin(al);
condition = a >= 0 & b ~= 0 & c ~= 0;
end

== matlab function Delta_Model_Separate/IKINE/MATLAB Function4 ==
  data: l1 input; condition output; l1 output; l2 output; xei output; yei output; zei output; xp output; yp output; zp output; al output; l2 input; xei input; yei input; zei input; xp input; yp input; zp input; a output; b output; al input; c output
function [condition, l1, l2, xei, yei, zei, xp, yp, zp, al, a, b, c] = condition(l1, l2, xei, yei, zei, xp, yp, zp, al)
a = 2*l2^2*xei^2 + 2*l2^2*xp^2 + 2*l2^2*yei^2 + 2*l2^2*yp^2 + 2*l1^2*zei^2 + 2*l2^2*zei^2 + 2*l1^2*zp^2 + 2*l2^2*zp^2 - 6*xei^2*xp^2 - 2*xei^2*yei^2 - 2*xei^2*yp^2 - 2*xp^2*yei^2 - 2*xp^2*yp^2 - 2*xei^2*zei^2 - 2*xei^2*zp^2 - 2*xp^2*zei^2 - 6*yei^2*yp^2 - 2*xp^2*zp^2 - 2*yei^2*zei^2 - 2*yei^2*zp^2 - 2*yp^2*zei^2 - 2*yp^2*zp^2 - 6*zei^2*zp^2 + 4*xei*xp^3 + 4*xei^3*xp + 4*yei*yp^3 + 4*yei^3*yp + 4*zei*zp^3 + 4*zei^3*zp - l1^4 - l2^4 - xei^4 - xp^4 - yei^4 - yp^4 - zei^4 - zp^4 + 2*l1^2*l2^2 - 4*l2^2*xei*xp - 4*l2^2*yei*yp - 4*l1^2*zei*zp - 4*l2^2*zei*zp + 2*l1^2*xei^2*cos(2*al) + 2*l1^2*xp^2*cos(2*al) - 2*l1^2*yei^2*cos(2*al) - 2*l1^2*yp^2*cos(2*al) + 4*xei*xp*yei^2 + 4*xei*xp*yp^2 + 4*xei*xp*zei^2 + 4*xei^2*yei*yp + 4*xei*xp*zp^2 + 4*xp^2*yei*yp + 4*yei*yp*zei^2 + 4*xei^2*zei*zp + 4*yei*yp*zp^2 + 4*xp^2*zei*zp + 4*yei^2*zei*zp + 4*yp^2*zei*zp - 4*l1^2*xei*xp*cos(2*al) + 4*l1^2*yei*yp*cos(2*al) - 8*xei*xp*yei*yp - 8*xei*xp*zei*zp - 8*yei*yp*zei*zp + 4*l1^2*xei*yei*sin(2*al) - 4*l1^2*xei*yp*sin(2*al) - 4*l1^2*xp*yei*sin(2*al) + 4*l1^2*xp*yp*sin(2*al);
b = xei^2*cos(al)^2 - 2*zei*zp + xp^2*cos(al)^2 + yei^2*sin(al)^2 + yp^2*sin(al)^2 + zei^2 + zp^2 - 2*xei*xp*cos(al)^2 + xei*yei*sin(2*al) - xei*yp*sin(2*al) - xp*yei*sin(2*al) + xp*yp*sin(2*al) - 2*yei*yp*sin(al)^2;
c = xei*cos(al) - xp*cos(al) + yei*sin(al) - yp*sin(al);
condition = a >= 0 & b ~= 0 & c ~= 0;
end
